simulink model "simulation_poursuite_discret"  (Simulink 7.6)
settings: Solver=ode45  StartTime=0  StopTime=30  RelTol=1e-3
values from neighbouring files (symbols this model uses):
  Te = 0.00001    (= 1e-05)    [PetitGain24V_discret.m]
undefined symbols (not defined in the file or in its folder): den_IMC, num_IMC
libraries: cstblocks x1
settings Model: Creator=Nicolas  LastModifiedBy=Igor

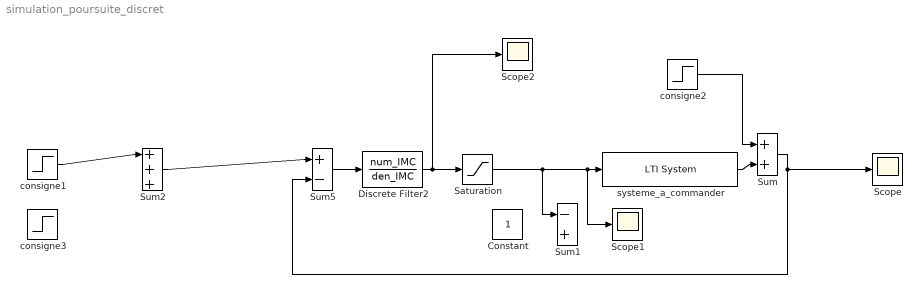
== system simulation_poursuite_discret ==
  Constant : Constant
  Discrete Filter2 : DiscreteFilter  Numerator=num_IMC  Denominator=den_IMC  SampleTime=Te
  Saturation : Saturate  UpperLimit=0.8  LowerLimit=0  SampleTime=Te
  Scope : Scope
      settings: TimeRange=35  YMin=0  YMax=35  MaxDataPoints=50000  SampleInput=on  SampleTime=Te
  Scope1 : Scope
      settings: TimeRange=5  YMin=0.1  YMax=1  MaxDataPoints=50000  SampleInput=on  SampleTime=Te
  Scope2 : Scope
      settings: TimeRange=0.1003764115432873  YMin=0.2  YMax=0.2011953551912569  SaveName=ScopeData2  MaxDataPoints=50000  SampleInput=on  SampleTime=Te
  Sum : Sum  Inputs=|++  SampleTime=Te
  Sum1 : Sum  Inputs=|-+  SampleTime=Te
  Sum2 : Sum  Inputs=|+++  SampleTime=Te
  Sum5 : Sum  Inputs=|+-  SampleTime=Te
  consigne1 : Step  After=18  SampleTime=Te
  consigne2 : Step  Time=3  SampleTime=Te
  consigne3 : Step  Time=5  After=6  SampleTime=Te
  systeme_a_commander : cstblocks/LTI System  SystemSampleTime=-1  sys=G_disc1  IC=[]
  wires:
  Sum5/1 -> Discrete Filter2/1
  systeme_a_commander/1 -> Sum/2
  Sum/1 -> Scope/1, Sum5/2
  Discrete Filter2/1 -> Saturation/1, Scope2/1
  Saturation/1 -> Sum1/1, systeme_a_commander/1, Scope1/1
  Sum2/1 -> Sum5/1
  consigne1/1 -> Sum2/1
  consigne2/1 -> Sum/1
